simulink library "ET3036TU_model_library_2021b"  (R2021b)
settings: Solver=VariableStepAuto  StartTime=0.0  StopTime=10.0  RelTol=1e-3
values from neighbouring files (symbols this model uses):
  Data =     [Data.mat]
  E_tol = 100    [run_test.m]
  Fnom = 50    [run_test.m]
  OverChargingProtection = 0    [run_test.m]
  simulation_mode = 2    [run_test.m]
  T_err = 60*60    (= 3600)    [run_test.m]
  Tsample = 60    [run_test.m]
  Vnom = sqrt(3)*230    [run_test.m]
undefined symbols (not defined in the file or in its folder): sigbuilder_block, sim_text
libraries: simulink x13, spsThreePhaseDynamicLoadLib x5, spsPower3phPhasorLib x3, eePowerMeasurement x2, spsThreePhaseVIMeasurementLib x2, spsThreePhaseSourceLib x2, spspowerguiLib x2, spsPower3phInstantaneousLib x1, spsThreePhaseSeriesRLCLoadLib x1, $bdroot x1
(part 1 of 2)
Description:
  | The following SIMULINK library is designed for the course "ET3036TU- PROJECT DESIGN FOR SUSTAINABLE ENERGY SYSTEMS". This is offered by EEMCS, TU Delft.
  | The following library was originally developed in R2020a and updated to 2020b. Contributors: N. K. Panda (n.k.panda@tudelft.nl), Simon Tindemans (s.h.tindemans@tudelft.nl)
settings Model: ModifiedComment=nkpanda -- 14 Nov 14:41:00 2023 -- Version2023.1 -- Updated to 2023b  Creator=Hazem  LastModifiedBy=nkpanda
settings Model: ModifiedHistory=|
  | nkpanda -- 14 Nov 14:41:00 2023 -- Version2023.1 -- Updated to 2023b
  | 
  | nkpanda -- Thu Dec 01 18:21:02 2022 -- Version 2.023160e+03 --updated bus meassurement icon
  | 
  | nkpanda -- Thu Dec 01 18:06:26 2022 -- Version 2.023150e+03
  | 
  | nkpanda -- Thu Dec 01 18:02:35 2022 -- Version 2.023140e+03 --renamed V2
  | 
  | nkpanda -- Mon Nov 28 16:04:20 2022 -- Version 2.023100e+03 -- meassurement channel updates
  | 
  | nkpanda -- Mon Nov 28 15:57:43 2022 -- Version 2022.10 (updated bus meassurement)
  | 
  | nkpanda -- Wed Nov 23 09:50:22 2022 -- Version 2.023500e+03
  | 
  | nkpanda -- Wed Nov 23 09:47:48 2022 -- Version 2022_updated_savedparam
  | 
  | nkpanda -- Upload version Tue Nov 15 14:46:24 2022 -- Version 2.022.4
  | 
  | nkpanda -- Tue Nov 15 14:32:50 2022 -- Version 2022.3
  | 
  | nkpanda -- Tue Nov 15 14:15:04 2022 -- Version 2022.2
  | 
  | nkpanda -- Tue Nov 15 13:41:17 2022 -- Version 2022.1
  | 
  | Original version: cc Hazem
  | Lates version : cc nkpanda
settings SolverCC: AlgebraicLoopSolver=TrustRegion
settings DebuggingCC: SFMachineParentedDataDiag=warning  ArithmeticOperatorsInVariantConditions=warning
settings SFSimCC: CustomCodeUndefinedFunction=UseInterfaceOnly

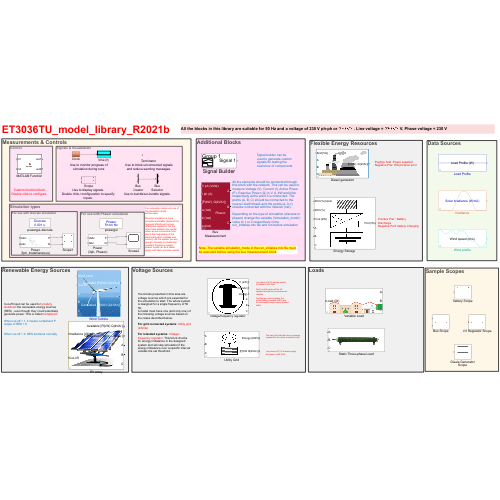
[thumbnail: Simulink's stored preview of the top-level diagram]
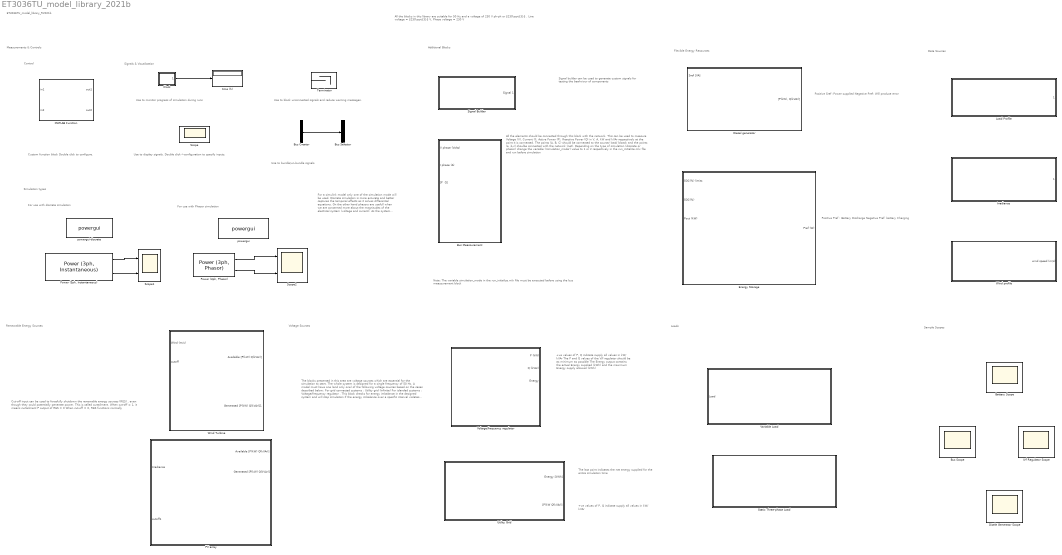
== system ET3036TU_model_library_2021b ==
  note: Note: The variable simulation_mode in the run_initialize.mlx file must be executed before using the bus meassurement block
  note: For a simulink model only one of the simulation mode
      | will be used.
      |
      | Discrete simulation is more accurate and better captures the temporal effects as it solves differential equations. On the other hand phasors are usefull when we are concerned more about the magnitudes of the electrical system (voltage and current). As the system you are going to develop is a balanced constant frequency system, phasor mode can be a faster option with fairly accurate results,
  note: Data Sources
  note: Additional Blocks
  note: Sample Scopes
  note: All the blocks in this library are suitable for 50 Hz and a voltage of 230 V ph-ph or $230\sqrt{3}$ . Line voltage = $230\sqrt{3}$ V, Phase voltage = 230 V
  note: +ve values of P, Q indicate supply
      | all values in kW/ kVAr
      |
      | The P and Q values of the V/f regulator should be as minimum as possible
      |
      | The Energy output contains the actual Energy supplied (kWh) and the maximum Energy supply allowed (kWh)
  note: All the elements should be connected through this block with the network. This can be used to measure Voltage (V), Current (I), Active Power (P), Reactive Power (Q) in V, A, kW and kVAr respectively at the point it is connected. The points (A, B, C) should be connected to the source/ load/ bloack and the points (a ,b,c) shoulbe connected with the network (net).
      |
      | Depending on the type of simulation (discrete or phasor) change the variable ('simulation_mode') value to 1 or 2 respectively in the run_initialize.mlx file and run before simulation
  note: Flexible Energy Resources
  note: Signals & Visualization
  note: Control
  note: Simulation types
  note: ET3036TU_model_library_R2021b
  note: The blocks presented in this area are voltage sources which are essential for the simulation to start. The whole system is designed for a single frequency of 50 Hz.
      | A model must have one (and only one) of the following voltage sources based on the cases described below:
      |
      | For grid connected systems : Utility grid (infinite)
      |
      | For islanded systems : Voltage/frequency regulator . This block checks for energy imbalance in the designed system and will stop simulation if the energy imbalance over a specific interval violates the set threshold.
  note: Loads
  note: Voltage Sources
  note: Custom function block
      | Double click to configure.
  note: Use to display signals.
      | Double click->configuration to specify inputs.
  note: Use to bundle\un-bundle signals.
  note: Use to block unconnected signals
      | and reduce warning messages.
  note: Measurements & Controls
  note: Renewable Energy Sources
  note: For use with Phasor simulation
  note: For use with discrete simulation
  note: Use to monitor progress of
      | simulation during runs
  note: +ve values of P, Q indicate supply
      | all values in kW/ kVAr
  note: The last point indicates the net energy supplied for the entire simulation time
  note: Positive Pref : Battery Discharge
      | Negative Pref: battery Charging
  note: Positive Sref :Power supplied
      | Negative Pref: Will produce error
  note: Signal builder can be used to generate custom signals for testing the beahviour of components
  note: Cut-off input can be used to forcefully shutdown the renewable energy sources (RES) , even though they could potentially generate power. This is called curtailment.
      |
      | When cut-off = 1, it means curtailment P output of RES = 0
      |
      | When cut-off = 0, RES functions normally
  Battery Scope : Scope
  Bus Creator : BusCreator  Inputs=2
  Bus Selector : BusSelector  OutputSignals=Active power P (W),Reactive power Q (var)
  "Bus Meassurement " : Subsystem  mask{SimModeSelect=simulation_mode, dispText=sim_text}
      mask prompts: SimModeSelect "Simulation mode"; dispText "Mode"
      mask init:
      | if SimModeSelect==1
      |     dispText = 'Discrete'
      | elseif SimModeSelect==2
      |     dispText = 'Phasor'
      | end
      mask Display:
      | color('white')
      | port_label('RConn',1,'a (net)')
      | port_label('RConn',2,'b (net)')
      | port_label('RConn',3,'c (net)')
      | port_label('LConn',1,'A')
      | port_label('LConn',2,'B')
      | port_label('LConn',3,'C')
      | 
      | 
      | port_label('output',1,'V ph (Volts)')
      | port_label('output',2,'I ph (A)')
      | port_label('output',3,'[P(kW), Q(kVAr)]')
      | 
      | get_param(gcb,'dispText')
      | 
      | fid = 'ssss'
      | fprintf('            %s \n \n \n \n ',dispText)
  Bus Scope : Scope  NumInputPorts=2
  Clock : Subsystem
  Diesel generator : Subsystem  mask(Controllable Power Plant){Snom=10, Vnom=Vnom, fnom=Fnom, Pfactor=1}
      mask prompts: Snom "Rated Power (kVA)"; Vnom "Rated Line  voltage (Vrms)"; fnom "Frequency (Hz)"; Pfactor "Power Factor (leading)"
      mask help: Implements a controllable (dispatchable) power plant with the required governer and excitation subsystems.
      mask Display: image('$imagefile'); % Use "Edit Image" on toolstrip to change.
  Disele Generator Scope : Scope
  Energy Storage : Subsystem  mask(Grid-connected Energy Storage (PQ Model)){Vn=Vnom, Fn=Fnom, PnomkW=10, kWh_Rated=1, Efficiency=100, LimitVec=[90 10], RechargeSOC=50, Precharge=100, autoRecharge=off, Initial_kWh_pc=35, PQvec=[0 0], ovrchargpro=OverChargingProtection}
      mask prompts: Vn "Nominal Line Voltage [Vrms]"; Fn "Nominal Frequency [Hz]"; PnomkW "Rated Power [kW]"; kWh_Rated "Rated Capacity [kWh]"; Efficiency "Overall System Efficiency [%]"; LimitVec "Upper/Lower Charge Limits [%]"; RechargeSOC "SOC to Recharge [%]"; Precharge "Recharge Rate [% of Rated Power]"; autoRecharge "Enable Auto-Recharge"; Initial_kWh_pc "Initial State-of-Charge [0-100%]"; PQvec "Initial Active/Reactive Cmds"; ovrchargpro "Enable over charging/ discharging protection (0: Disable, 1: Enable)"
      mask help:
      | The energy storage block models a generic grid-connected energy storage system (ESS), most commonly a battery system. This is a system-level model that does not contain any power electronics, but is useful for load flow, phasor, and hybrid phasor-EMT simulations. The inputs to this block are the commanded active and reactive power of the ESS.
      |
      | Note: Positive cmd indicates discharging (supply), negative cmd indicates charging (load).
      | Note: The initial active/reactive power commands must be specified for use for Load Flow analysis.
      mask init:
      | % Calculate Initial Conditions
      | Pnom = PnomkW*1e3;
      | P0 = -PQvec(1);  Q0 = -PQvec(2);
      | if abs(P0) > Pnom
      |     P0 = sign(P0)*Pnom;
      | end
      | 
      | % Calculate Q0 given Reactive Power Capability Curve
      | Qlim = sqrt(Pnom^2 - P0^2);
      | if Qlim > abs(Q0)
      |     Q0 = sign(Q0)*Qlim;
      | end
      | 
      | UpChrgLim = LimitVec(1);
      | LowChrgLim = LimitVec(2);
      | if Initial_kWh_pc > UpChrgLim && P0 < 0
      |     P0 = 0; Q0 = 0;
      | elseif Initial_kWh_pc < LowChrgLim && P0 > 0
      |     P0 = 0; Q0 = 0;
      | end
      mask DialogControl Container7 Prompt: Grid Connection Properties
      mask DialogControl Container11 Prompt: Charge/Discharge Controls
      mask DialogControl Container12 Prompt: Initial Conditions
      mask Display: image('$imagefile'); % Use "Edit Image" on toolstrip to change.
  Irradiance : Subsystem  mask(Irradiance profile){}
      mask help:
      | Automatically loads irradiance values from the local file 'Data.mat' (variable Data.solar).
      |
      | Expects hourly input irradiance values (W/m2).
      mask init:
      | load Data
      mask Display:
      | plot(Data.solar.hour(1:24),Data.solar.direct(1:24)+Data.solar.diffuse(1:24))
      | 
      | color('blue')
      | disp('Solar Irradiance (W/m2)')
  Load Profile : Subsystem
      mask init:
      | load Data
      mask DialogControl DescGroupVar Prompt: Load Profile
      mask DialogControl DescTextVar Prompt: Automatically loads Consumption values from the local file 'Data.mat' (variable Data.varload).
      mask DialogControl Control2 Prompt: Expects per-minute active power consumption values (W).
      mask Display:
      | plot(Data.varload.minute(120:150),Data.varload.load(120:150))
      | color('black')
      | disp('Load Profile (W)')
  MATLAB Function : MATLAB Function  TreatAsAtomicUnit=on
  "PV array " : Subsystem  mask(PV farm){Efficiency=0.2, Area=100, Vnom=Vnom, fnom=Fnom}
      mask prompts: Efficiency "Total efficiency (fraction)"; Area "Area (m2)"; Vnom "Rated Line voltage (Vrms)"; fnom "Rated frequency (Hz):"
      mask help: The product of the efficiency, the area covered by the PV farm and the irradiance in W/m2 will give you the power generated by the PV farm.
      mask Display:
      | color('white')
      | image(imread('pv.jpg'))
      | 
      | color('black')
      | port_label('RConn',1,'A')
      | port_label('RConn',2,'B')
      | port_label('RConn',3,'C')
      | port_label('output',1,'Available [P(kW) Q(kVAr)]')
      | port_label('output',2,'Generated [P(kW) Q(kVAr)]')
      | 
      | port_label('input',1,'Irradiance (W/m2)')
      | port_label('input',2,'Cut-off')
  "Power (3ph, Instantaneous)" : spsPower3phInstantaneousLib/Power (3ph, Instantaneous)
  "Power (3ph, Phasor)" : spsPower3phPhasorLib/Power (3ph, Phasor)
      settings: SourceProductBaseCode=PS
  Scope : Scope  NumInputPorts=2
  Scope1 : Scope  NumInputPorts=2
  Scope2 : Scope  NumInputPorts=2
  Signal Builder : Subsystem  Tag=STV Subsys  LoadFcn=sigbuilder_block('load');  StartFcn=sigbuilder_block('start');  StopFcn=sigbuilder_block('stop');  ClipboardFcn=sigbuilder_block('clipboard');  mask(Sigbuilder block){tuvar=[0:10]}
      mask help: Simulink:masks:SigbuilderBlock_MD
      mask init:
      | if ~strcmp(get_param(bdroot(gcbh),'SimulationStatus'),'stopped') tuvar = sigbuilder_block('maskInit'); end
      settings: CopyFcn=sigbuilder_block('copy');  DeleteFcn=sigbuilder_block('delete');  ModelCloseFcn=sigbuilder_block('modelClose');  PreSaveFcn=sigbuilder_block('preSave');  PauseFcn=sigbuilder_block('pause');  ContinueFcn=sigbuilder_block('continue');  NameChangeFcn=sigbuilder_block('namechange');  OpenFcn=sigbuilder_block('open',[437.6 199.2 550.4 400 ]);  CloseFcn=sigbuilder_block('close');
      mask Display: plot(0, 0, 100, 100,[2, 2, 32, 32, 2], [68, 8, 8, 68, 68],[32, 2], [38, 38], [32, 19, 2],[53, 60, 44], [32, 17, 17, 2],[16, 16, 31, 31]);txt = getActiveGroup(gcbh);text(2, 100, txt,'verticalAlignment', 'top');
  Static Three-phase Load : Subsystem  mask(Static Three-phase Load){Vnom=Vnom, fnom=Fnom, Prated=10}
      mask prompts: Vnom "Nominal Line Voltage Vn (Vrms)"; fnom "Nominal frequency fn (Hz):"; Prated "Active power P (kW):"
      mask help:
      | Implements a three-phase resistive load.
      |
      | Adjust nominal voltage and frequency according to system configuration.
      |
      | Specify rated power consumption.
      mask Display: image(imread('Res.jpg'))
  Terminator : Terminator
  Utility Grid : Subsystem  mask(Utility Distribution Substation){Vnommask=Vnom, Fnommask=Fnom}
      mask prompts: Vnommask "Grid Line voltage (Vrms)"; Fnommask "Nominal frequency (Hz):"
      mask help:
      | Implements a grid connection with finite capacity.
      |
      | Supports two-way power flow, set voltages and frequency according to system configuration.
      |
      | Adjust Nominal Power.
      mask Display: image('$imagefile'); % Use "Edit Image" on toolstrip to change.
  V/f Regulator Scope : Scope
  Variable Load : Subsystem  mask(Variable Load (PQ Model)){Vn=Vnom, Fn=Fnom, PF=1, Load0=0}
      mask prompts: Vn "Nominal Line Voltage [Vrms]"; Fn "Nominal Frequency [Hz]"; PF "Power Factor [0 to 1]"; Load0 "Initial Load [W]"
      mask help:
      | The Variable Load block is a lumped approximation for a distribution feeder. For non-unity power factor loads, the input (active power) is scaled accordingly to generate a desired load.
      |
      | Note: The initial input load must be specified for use for Load Flow analysis.
      mask init:
      | P0 = Load0;
      | Q0 = Load0*sqrt(1/PF-1);
      mask Display:
      | image('house.png')
      | color('black')
      | port_label('input',1,'Load (W)')
      | port_label('Rconn',1,'A')
      | port_label('Rconn',2,'B')
      | port_label('Rconn',3,'C')
  Voltage/frequency regulator : Subsystem  mask{E_max=E_tol, Terr=T_err, Vnommask=Vnom, Fnommask=Fnom}
      mask prompts: E_max "Energy error tolerance  (Wh)"; Terr "Error re-set time-period (seconds)"; Vnommask "Nominal Line Voltage (Vrms)"; Fnommask "Nominal Frequency (Hz)"
      mask Display: image('$imagefile'); % Use "Edit Image" on toolstrip to change.
  "Wind Turbine " : Subsystem  mask{Unom=15, Umax=25, Umin=5, Pselect=1: Simple Cubic Power, fnom=Fnom, Vnom=Vnom, Pnom=20, rp=5, Cp=16/27, rho=1.225, Uvec=1:1:30, Pvec=[0,0,0,0,21359.3750000000,58193.5000000000,104316.125000000,157104.500000000,213935.875000000,272187.500000000,329236.625000000,382460.500000000,429236.375000000,466941.500000000,492953.125000000,500000,500000,500000,500000,500000,500000,500000,500000,500000,500000,0,0,0,0,0], Tp=1, Tq=0.1, ReactP=0}
      mask prompts: Unom "Nominal Wind Speed [m/s]"; Umax "Maximum Operating Wind [m/s]"; Umin "Minimum Operating Wind [m/s]"; Pselect "Wind Turbine Power Model"; fnom "Nominal frequency (Hz):"; Vnom "Nominal phae-to-phase voltage (Vrms)"; Pnom "Nominal Power, [kW]"; rp "Blade Radius, r [m]"; Cp "Performance Coefficient, Cp"; rho "Air Density, rho [kg/m^3]"; Uvec "Wind Vec [m/s]"; Pvec "Power Vec [W]"; Tp "Active Power Dynamics, Tp [s]"; Tq "Reactive Power Dynamics, Tq [s]"; ReactP "Reactive Power Percentage [%]"
      mask help:
      | Simple Wind Turbine that serves as an Active and Reactive Power Source depending on the Wind Power Curve.
      |
      | The Wind Turbine Power Curve can be defined by one of three models:
      | 1: Simple cubic power curve
      | 2: Physical wind turbine parameters
      | 3: Look-up table (from a wind turbine data sheet).
      |
      | Cutoff takes value 1 or 0. 1 denotes manual forced cut-off od wind power generation even though potnetial wind power is available
      | The 'General' and 'Dynamics' tabs apply to all models.
      mask init:
      | A = pi*rp^2;
      | 
      | if Pselect == 1,
      |     Pmax = Pnom*1e3;
      | elseif Pselect == 2,
      |     Pmax = 1/2*rho*Cp*A*Umax^3;
      | else
      |     Pmax = max(Pvec);
      | end
      | Qmax = (ReactP/100)*Pmax;
      mask TypeOptions Pselect: 1: Simple Cubic Power | 2: Physical parameters | 3: Look-up Fit
      mask DialogControl Container4 Prompt: General
      mask DialogControl Container16 Prompt: Turbine
      mask DialogControl Container10 Prompt: Electrical
      mask DialogControl Container12 Prompt: 1: Cubic
      mask DialogControl Container9 Prompt: 2: Physical
      mask DialogControl Container7 Prompt: 3: Lookup
      mask DialogControl Container8 Prompt: Dynamics
      mask Display:
      | image(imread('eolienne.bmp'))
      | 
      | color('white')
      | port_label('LConn',1,'A')
      | port_label('LConn',2,'B')
      | port_label('LConn',3,'C')
      | 
      | port_label('output',1,'Available [P(kW) Q(kVAr)]')
      | port_label('output',2,'Generated [P(kW) Q(kVAr)]')
      | port_label('input',1,'Wind (m/s)')
      | port_label('input',2,'Cut-off')
  Wind profile : Subsystem  mask(Wind profile){}
      mask help:
      | Automatically loads wind speeds from the local file 'Data.mat' (variable Data.wind).
      |
      | Expects hourly input wind speeds (m/s).
      mask init:
      | load Data
      mask Display:
      | plot(Data.wind.hour(1:24),Data.wind.speed(1:24))
      | color('black')
      | disp('Wind speed (m/s)')
  powergui : spspowerguiLib/powergui  Priority=1  SimulationMode=Phasor  SampleTime=50e-6  frequency=Fnom  Iterations=50  frequencyindice=60  Pbase=100e6  ErrMax=1e-4  UnitsV=kV  UnitsW=MW  buscounter=0  FunctionMessages=off  echomessages=off  EnableUseOfTLC=off  CurrentSourceSwitches=off  DisableSnubberDevices=off  DisableRonSwitches=off  DisableVfSwitches=off  DisplayEquations=off  AutomaticDiscreteSolvers=off  SolverType=Tustin/Backward Euler (TBE)  Interpol=off  ExternalGateDelay=off  methode=off  Ts=100  x0status=blocks  SPID=on  SwTol=0  HookPort=off  NonlinearTolerance=1e-4  nMaxIteration=100  ContinueOnMaxIteration=off  RestoreLinks=warning  ResistiveCurrentMeasurement=off  Frange=[0:2:500]  Ylog=off  Xlog=on  ShowGrid=off  save=off  variable=ZData  structure=0  ZoomFFT=off  StartTime=0.0  cycles=1  DisplayStyle=1  fundamental=60  FreqAxis=off  MaxFrequency=1000  frequencyindicesteady=1  RmsSteady=1  display=off
  powergui-discrete : spspowerguiLib/powergui  Priority=1  SimulationMode=Discrete  SampleTime=1e-3  frequency=60  Iterations=50  frequencyindice=60  Pbase=100e6  ErrMax=1e-4  UnitsV=kV  UnitsW=MW  buscounter=0  FunctionMessages=off  echomessages=off  EnableUseOfTLC=off  CurrentSourceSwitches=off  DisableSnubberDevices=off  DisableRonSwitches=off  DisableVfSwitches=off  DisplayEquations=off  AutomaticDiscreteSolvers=off  SolverType=Tustin/Backward Euler (TBE)  Interpol=off  ExternalGateDelay=off  methode=off  Ts=100  x0status=blocks  SPID=on  SwTol=0  HookPort=off  NonlinearTolerance=1e-4  nMaxIteration=100  ContinueOnMaxIteration=off  RestoreLinks=warning  ResistiveCurrentMeasurement=off  Frange=[0:2:500]  Ylog=off  Xlog=on  ShowGrid=off  save=off  variable=ZData  structure=0  ZoomFFT=off  StartTime=0.0  cycles=1  DisplayStyle=1  fundamental=60  FreqAxis=off  MaxFrequency=1000  frequencyindicesteady=1  RmsSteady=1  display=off
  time (h) : Display
      settings: Format=bank
  wires:
  "Power (3ph, Phasor)"/1 -> Scope2/1
  "Power (3ph, Phasor)"/2 -> Scope2/2
  "Power (3ph, Instantaneous)"/1 -> Scope1/1
  "Power (3ph, Instantaneous)"/2 -> Scope1/2
  Clock/1(" ") -> time (h)/1
  Bus Creator/1 -> Bus Selector/1

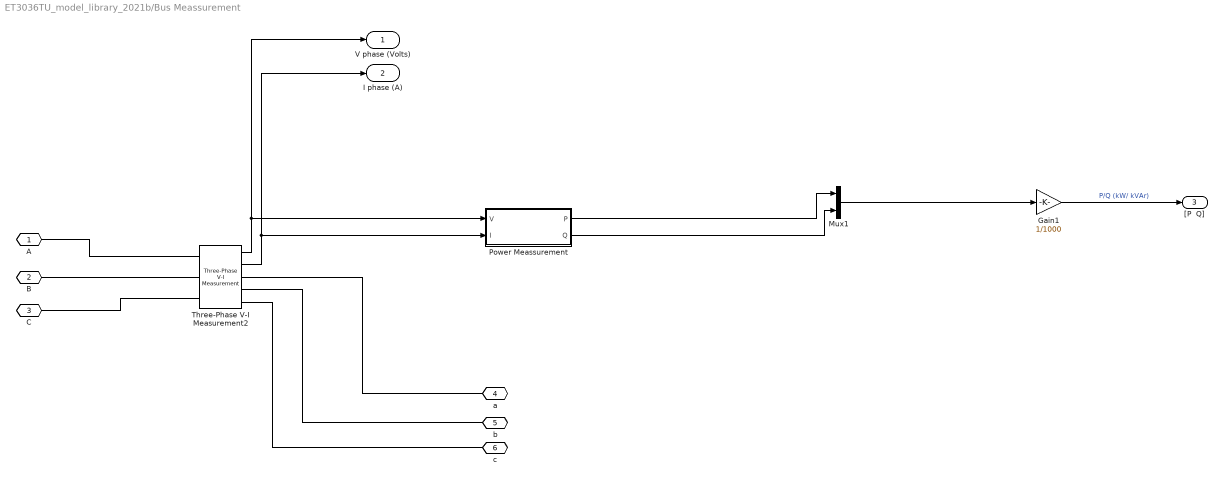
== system ET3036TU_model_library_2021b/Bus Meassurement  ==
  Gain1 : Gain  Gain=1/1000
  Mux1 : Mux  Inputs=2
  Power Meassurement : Subsystem  Variant=on
  Three-Phase V-I Measurement2 : spsThreePhaseVIMeasurementLib/Three-Phase V-I Measurement  VoltageMeasurement=phase-to-ground  SetLabelV=off  LabelV=Vabc  Vpu=off  VpuLL=off  CurrentMeasurement=yes  SetLabelI=off  LabelI=Iabc  Ipu=off  Pbase=100e6  Vbase=500e3  OutputType=Complex  PhasorSimulation=off  PSBequivalent=0
  A : PMIOPort  Side=Left
  B : PMIOPort  Port=2  Side=Left
  C : PMIOPort  Port=3  Side=Left
  a : PMIOPort  Port=4  Side=Right
  b : PMIOPort  Port=5  Side=Right
  c : PMIOPort  Port=6  Side=Right
  V phase (Volts) : Outport
  I phase (A) : Outport  Port=2
  "[P  Q]" : Outport  Port=3
  wires:
  Gain1/1 -> "[P  Q]"/1  "P/Q (kW/ kVAr)"
  Mux1/1 -> Gain1/1
  Three-Phase V-I Measurement2/2 -> I phase (A)/1, Power Meassurement/2(I)
  Three-Phase V-I Measurement2/1 -> V phase (Volts)/1, Power Meassurement/1(V)
  Power Meassurement/2(Q) -> Mux1/2
  Power Meassurement/1(P) -> Mux1/1
  connections:
  Three-Phase V-I Measurement2/LConn3 -- C/RConn1
  B/RConn1 -- Three-Phase V-I Measurement2/LConn2
  A/RConn1 -- Three-Phase V-I Measurement2/LConn1
  Three-Phase V-I Measurement2/RConn1 -- a/RConn1
  Three-Phase V-I Measurement2/RConn2 -- b/RConn1
  Three-Phase V-I Measurement2/RConn3 -- c/RConn1

== system ET3036TU_model_library_2021b/Clock ==
  Clock : Clock
  Gain : Gain  Gain=1/(60*60)
  " " : Outport  VectorParamsAs1DForOutWhenUnconnected=off
  wires:
  Gain/1 -> " "/1
  Clock/1 -> Gain/1

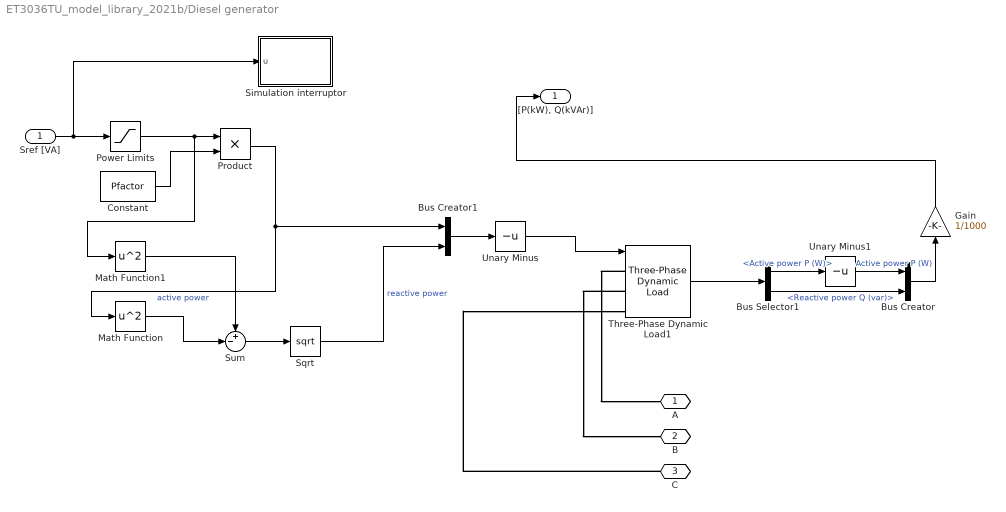
== system ET3036TU_model_library_2021b/Diesel generator ==
  Sref [VA] : Inport
  Bus Creator : BusCreator  Inputs=2
  Bus Creator1 : BusCreator  Inputs=2
  Bus Selector1 : BusSelector  OutputSignals=Active power P (W),Reactive power Q (var)
  Constant : Constant  Value=Pfactor
  Gain : Gain  Gain=1/1000
  Math Function : Math  Operator=square  SignedPower=on  SaturateOnIntegerOverflow=on
  Math Function1 : Math  Operator=square  SignedPower=on  SaturateOnIntegerOverflow=on
  Power Limits : Saturate  UpperLimit=Snom*1e3  LowerLimit=0
  Product : Product
  Simulation interruptor : MATLAB Function  TreatAsAtomicUnit=on
  Sqrt : Sqrt  SaturateOnIntegerOverflow=on
  Sum : Sum  Inputs=+-|
  Three-Phase Dynamic Load1 : spsThreePhaseDynamicLoadLib/Three-Phase Dynamic Load  NominalVoltage=[Vnom fnom]  ActiveReactivePowers="[ 0  0]"  PositiveSequence=[Vnom 0]  ExternalControl=on  NpNq=[1.3 2]  TimeConstants="[0  0  0  0]"  MinimumVoltage=0.7  Tfilter=1e-4  LoadFlowParameters=[4,0,0,0,0]
      settings: SourceProductBaseCode=PS
  Unary Minus : UnaryMinus
  Unary Minus1 : UnaryMinus
  A : PMIOPort  Side=Left
  B : PMIOPort  Port=2  Side=Left
  C : PMIOPort  Port=3  Side=Left
  "[P(kW), Q(kVAr)]" : Outport  VectorParamsAs1DForOutWhenUnconnected=off
  wires:
  Gain/1 -> "[P(kW), Q(kVAr)]"/1
  Constant/1 -> Product/2
  Math Function1/1 -> Sum/1
  Math Function/1 -> Sum/2
  Product/1 -> Math Function/1, Bus Creator1/1  "active power"
  Sref [VA]/1 -> Power Limits/1, Simulation interruptor/1(u)
  Sum/1 -> Sqrt/1
  Power Limits/1 -> Math Function1/1, Product/1
  Sqrt/1 -> Bus Creator1/2  "reactive power"
  Bus Selector1/2 -> Bus Creator/2  "<Reactive power Q (var)>"
  Three-Phase Dynamic Load1/1 -> Bus Selector1/1
  Bus Selector1/1 -> Unary Minus1/1  "<Active power P (W)>"
  Unary Minus1/1 -> Bus Creator/1  "Active power P (W)"
  Bus Creator/1 -> Gain/1
  Bus Creator1/1 -> Unary Minus/1
  Unary Minus/1 -> Three-Phase Dynamic Load1/1
  connections:
  C/RConn1 -- Three-Phase Dynamic Load1/LConn3
  Three-Phase Dynamic Load1/LConn2 -- B/RConn1
  Three-Phase Dynamic Load1/LConn1 -- A/RConn1

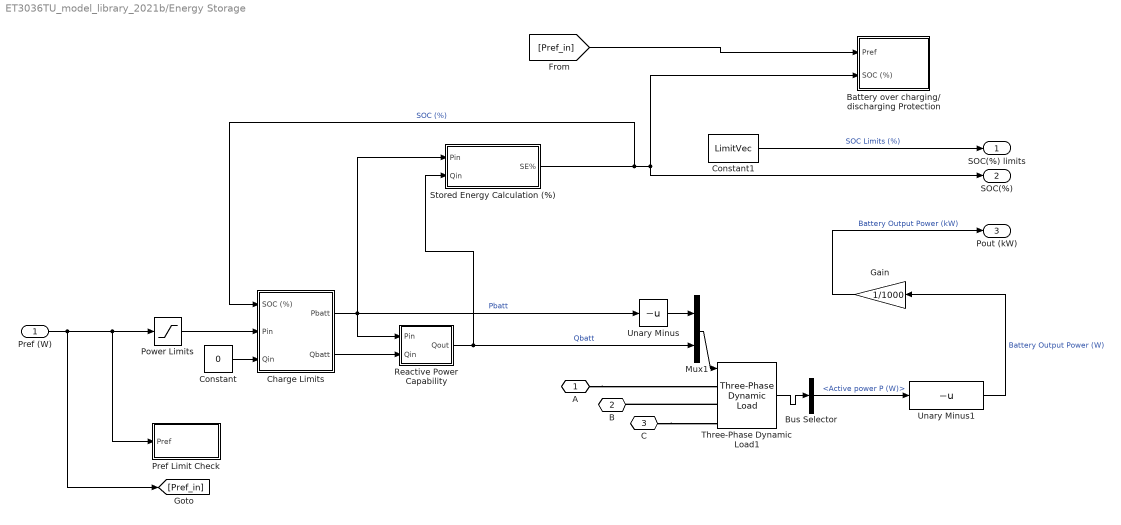
== system ET3036TU_model_library_2021b/Energy Storage ==
  Pref (W) : Inport
  Battery over charging/ discharging Protection : Subsystem
  Bus Selector : BusSelector  OutputSignals=Active power P (W)
  Charge Limits : Subsystem
  Constant : Constant  Value=0
  Constant1 : Constant  Value=LimitVec
  Gain : Gain  Gain=1/1000
  Mux1 : Mux  Inputs=2
  Power Limits : Saturate  UpperLimit=Pnom  LowerLimit=-Pnom
  Pref Limit Check : Subsystem
  Reactive Power Capability : Subsystem
  Stored Energy Calculation (%) : Subsystem
  Three-Phase Dynamic Load1 : spsThreePhaseDynamicLoadLib/Three-Phase Dynamic Load  NominalVoltage=[Vn Fn]  ActiveReactivePowers="[ 0  0]"  PositiveSequence=[Vn 0]  ExternalControl=on  NpNq=[1.3 2]  TimeConstants="[0  0  0  0]"  MinimumVoltage=0.7  Tfilter=1e-4  LoadFlowParameters=[4,0,0,0,0]
      settings: SourceProductBaseCode=PS
  Unary Minus : UnaryMinus
  Unary Minus1 : UnaryMinus
  A : PMIOPort  Side=Right
  B : PMIOPort  Port=2  Side=Right
  C : PMIOPort  Port=3  Side=Right
  SOC(%) limits : Outport  VectorParamsAs1DForOutWhenUnconnected=off
  SOC(%) : Outport  Port=2  VectorParamsAs1DForOutWhenUnconnected=off
  Pout (kW) : Outport  Port=3  VectorParamsAs1DForOutWhenUnconnected=off
  wires:
  Constant1/1 -> SOC(%) limits/1  "SOC Limits (%)"
  [Pref_in] -> Battery over charging/ discharging Protection/1(Pref)
  Gain/1 -> Pout (kW)/1  "Battery Output Power (kW)"
  Unary Minus1/1 -> Gain/1  "Battery Output Power (W)"
  Bus Selector/1 -> Unary Minus1/1  "<Active power P (W)>"
  Charge Limits/2(Qbatt) -> Reactive Power Capability/2(Qin)
  Constant/1 -> Charge Limits/3(Qin)
  Power Limits/1 -> Charge Limits/2(Pin)
  Charge Limits/1(Pbatt) -> Reactive Power Capability/1(Pin), Unary Minus/1, Stored Energy Calculation (%)/1(Pin)  "Pbatt"
  Stored Energy Calculation (%)/1(SE%) -> Charge Limits/1(SOC (%)), SOC(%)/1, Battery over charging/ discharging Protection/2(SOC (%))  "SOC (%)"
  Pref (W)/1 -> Power Limits/1, Pref Limit Check/1(Pref), [Pref_in]
  Reactive Power Capability/1(Qout) -> Mux1/2, Stored Energy Calculation (%)/2(Qin)  "Qbatt"
  Three-Phase Dynamic Load1/1 -> Bus Selector/1
  Mux1/1 -> Three-Phase Dynamic Load1/1
  Unary Minus/1 -> Mux1/1
  connections:
  A/RConn1 -- Three-Phase Dynamic Load1/LConn1
  C/RConn1 -- Three-Phase Dynamic Load1/LConn3
  Three-Phase Dynamic Load1/LConn2 -- B/RConn1

== system ET3036TU_model_library_2021b/Irradiance ==
  Add : Sum
  Add1 : Sum
  Clock1 : Clock
  Constant1 : Constant
  Diffuse irradiance series : Lookup_n-D  NumberOfTableDimensions=1  BreakpointsForDimension1=Data.solar.hour  BeginIndexSearchUsingPreviousIndexResult=on  Table=Data.solar.diffuse  InternalRulePriority=Speed  RndMeth=Simplest  InputSameDT=on
  Direct irradiance series : Lookup_n-D  NumberOfTableDimensions=1  BreakpointsForDimension1=Data.solar.hour  BeginIndexSearchUsingPreviousIndexResult=on  Table=Data.solar.direct  InternalRulePriority=Speed  RndMeth=Simplest  InputSameDT=on
  Second-->Hour : Gain  Gain=1/(60*60)
  " " : Outport  VectorParamsAs1DForOutWhenUnconnected=off
  wires:
  Constant1/1 -> Add/2
  Add/1 -> Direct irradiance series/1, Diffuse irradiance series/1  "Simulation hour"
  Clock1/1 -> Second-->Hour/1
  Second-->Hour/1 -> Add/1
  Diffuse irradiance series/1 -> Add1/1
  Direct irradiance series/1 -> Add1/2
  Add1/1 -> " "/1  "Simulation hour"

== system ET3036TU_model_library_2021b/Load Profile ==
  Add : Sum
  Clock1 : Clock
  Constant1 : Constant
  Second-->Minute : Gain  Gain=1/(60)
  load profile series : Lookup_n-D  NumberOfTableDimensions=1  BreakpointsForDimension1=Data.varload.minute  BeginIndexSearchUsingPreviousIndexResult=on  Table=Data.varload.load  InternalRulePriority=Speed  RndMeth=Simplest  InputSameDT=on
  " " : Outport  VectorParamsAs1DForOutWhenUnconnected=off
  wires:
  Constant1/1 -> Add/2
  Add/1 -> load profile series/1  "Minute"
  load profile series/1 -> " "/1
  Clock1/1 -> Second-->Minute/1
  Second-->Minute/1 -> Add/1

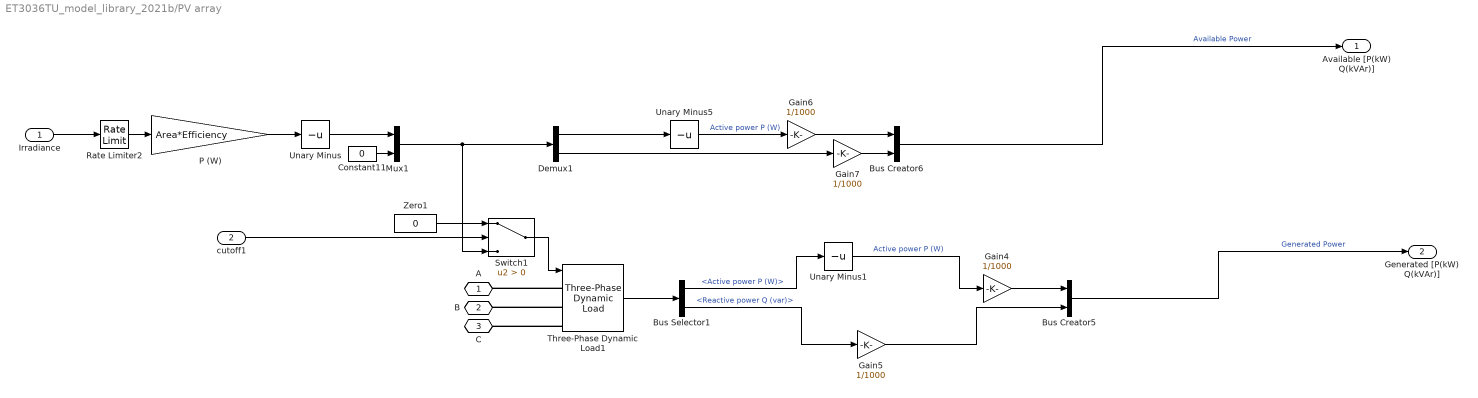
== system ET3036TU_model_library_2021b/PV array  ==
  Irradiance : Inport
  cutoff1 : Inport  Port=2
  Bus Creator5 : BusCreator  Inputs=2
  Bus Creator6 : BusCreator  Inputs=2
  Bus Selector1 : BusSelector  OutputSignals=Active power P (W),Reactive power Q (var)
  Constant11 : Constant  Value=0
  Demux1 : Demux  Outputs=2
  Gain{4..7} (4 alike) : Gain  Gain=1/1000
  Mux1 : Mux  Inputs=2
  P (W) : Gain  Gain=Area*Efficiency
  Rate Limiter2 : RateLimiter  RisingSlewLimit=1e4  FallingSlewLimit=-1e4  SampleTimeMode=inherited
  Switch1 : Switch  Criteria=u2 > Threshold
  Three-Phase Dynamic Load1 : spsThreePhaseDynamicLoadLib/Three-Phase Dynamic Load  NominalVoltage=[Vnom fnom]  ActiveReactivePowers="[ 0  0]"  PositiveSequence=[Vnom 0]  ExternalControl=on  NpNq=[1.3 2]  TimeConstants="[0  0  0  0]"  MinimumVoltage=0.7  Tfilter=1e-4  LoadFlowParameters=[4,0,0,0,0]
      settings: SourceProductBaseCode=PS
  Unary Minus : UnaryMinus
  Unary Minus1 : UnaryMinus
  Unary Minus5 : UnaryMinus
  Zero1 : Constant  Value=0  OutDataTypeStr=Inherit: Inherit via back propagation
  A : PMIOPort  Side=Right
  B : PMIOPort  Port=2  Side=Right
  C : PMIOPort  Port=3  Side=Right
  Available [P(kW) Q(kVAr)] : Outport  VectorParamsAs1DForOutWhenUnconnected=off
  Generated [P(kW) Q(kVAr)] : Outport  Port=2  VectorParamsAs1DForOutWhenUnconnected=off
  wires:
  Zero1/1 -> Switch1/1
  cutoff1/1 -> Switch1/2
  Mux1/1 -> Switch1/3, Demux1/1
  Switch1/1 -> Three-Phase Dynamic Load1/1
  Bus Creator6/1 -> Available [P(kW) Q(kVAr)]/1  "Available Power"
  Gain7/1 -> Bus Creator6/2
  Unary Minus5/1 -> Gain6/1  "Active power P (W)"
  Demux1/2 -> Gain7/1
  Gain6/1 -> Bus Creator6/1
  Demux1/1 -> Unary Minus5/1
  Gain5/1 -> Bus Creator5/2
  Gain4/1 -> Bus Creator5/1
  Bus Selector1/2 -> Gain5/1  "<Reactive power Q (var)>"
  Three-Phase Dynamic Load1/1 -> Bus Selector1/1
  Unary Minus1/1 -> Gain4/1  "Active power P (W)"
  Bus Selector1/1 -> Unary Minus1/1  "<Active power P (W)>"
  Irradiance/1 -> Rate Limiter2/1
  P (W)/1 -> Unary Minus/1
  Unary Minus/1 -> Mux1/1
  Constant11/1 -> Mux1/2
  Rate Limiter2/1 -> P (W)/1
  Bus Creator5/1 -> Generated [P(kW) Q(kVAr)]/1  "Generated Power"
  connections:
  Three-Phase Dynamic Load1/LConn3 -- C/RConn1
  Three-Phase Dynamic Load1/LConn1 -- A/RConn1
  Three-Phase Dynamic Load1/LConn2 -- B/RConn1

== system ET3036TU_model_library_2021b/Signal Builder ==
  Demux : Demux  Tag=STV Demux  Outputs=1
      settings: DisplayOption=none
  FromWs : FromWorkspace  Tag=STV FromWs  VariableName=tuvar
      SigBuilderData=|
      | common.afterFinalStr = 'Extrapolate'
      | common.sampleTime = 0
      | dataSet.timeRange = [0 10]
      | dataSet.name = 'Group 1'
      | sbobj.Groups.Name = 'Group 1'
      | sbobj.Groups.Signals.Name = 'Signal 1'
      | sbobj.Groups.Signals.XData = [0 4 4 6 6 10]
      | sbobj.Groups.Signals.YData = [0 0 1 1 0 0]
  Signal 1 : Outport  Tag=STV Outport
  wires:
  Demux/1 -> Signal 1/1
  FromWs/1 -> Demux/1

== system ET3036TU_model_library_2021b/Static Three-phase Load ==
  Three-Phase Series RLC Load : spsThreePhaseSeriesRLCLoadLib/Three-Phase Series RLC Load  LConnTagsString=A|B|C  Configuration=Y (grounded)  NominalVoltage=Vnom  Vabc=[1e3 1e3 1e3]  Vabcp=[1e3 1e3 1e3]  NominalFrequency=fnom  UnbalancedPower=off  ActivePower=Prated*1e3  InductivePower=100  CapacitivePower=100  Pabc=[10e3 9e3 11e3]  QLabc=[100 90 110]  QCabc=[100 90 110]  Pabcp=[10e3 9e3 11e3]  QLabcp=[100 90 110]  QCabcp=[100 90 110]  Measurements=None  LoadType=constant Z
  A : PMIOPort  Side=Left
  B : PMIOPort  Port=2  Side=Left
  C : PMIOPort  Port=3  Side=Left
  connections:
  Three-Phase Series RLC Load/LConn2 -- B/RConn1
  C/RConn1 -- Three-Phase Series RLC Load/LConn3
  A/RConn1 -- Three-Phase Series RLC Load/LConn1

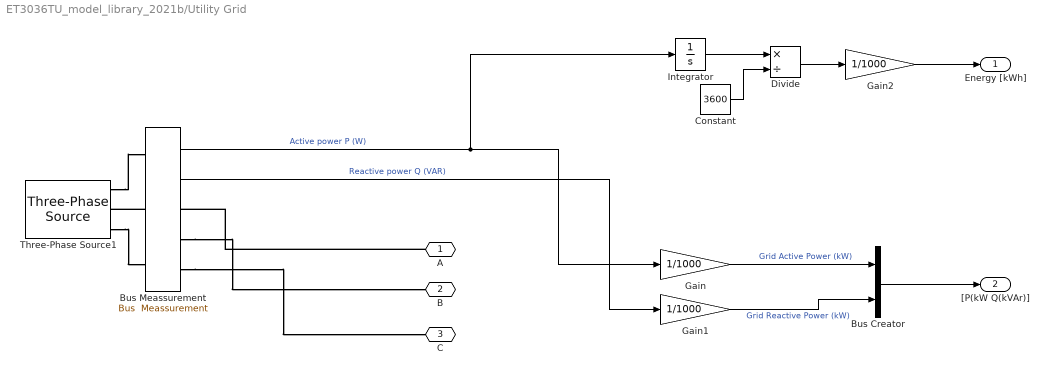
== system ET3036TU_model_library_2021b/Utility Grid ==
  Bus Creator : BusCreator  Inputs=2
  "Bus Meassurement " : $bdroot/Voltage//frequency regulator/Bus  Meassurement 
  Constant : Constant  Value=3600
  Divide : Product  Inputs=*/
  Gain : Gain  Gain=1/1000
  Gain1 : Gain  Gain=1/1000
  Gain2 : Gain  Gain=1/1000
  Integrator : Integrator
  Three-Phase Source1 : spsThreePhaseSourceLib/Three-Phase Source  InternalConnection=Yg  VoltagePhases=off  Voltage=Vnommask  PhaseAngle=0  Voltage_phases=[25e3 25e3 25e3]/sqrt(3)  PhaseAngles_phases=[0 -120 +120]  Frequency=Fnommask  NonIdealSource=off  SpecifyImpedance=off  Resistance=0.8929  Inductance=16.58e-3  ShortCircuitLevel=100e6  BaseVoltage=25e3  XRratio=7  BusType=swing  Pref=10e3  Qref=0  Prefabc=[10e3, 10e3, 10e3]  Qrefabc=[0, 0, 0]  Qmin=-inf  Qmax=inf
  A : PMIOPort  Side=Left
  B : PMIOPort  Port=2  Side=Left
  C : PMIOPort  Port=3  Side=Left
  Energy [kWh] : Outport  VectorParamsAs1DForOutWhenUnconnected=off
  "[P(kW Q(kVAr)]" : Outport  Port=2
  wires:
  Gain/1 -> Bus Creator/1  "Grid Active Power (kW)"
  Bus Creator/1 -> "[P(kW Q(kVAr)]"/1
  Constant/1 -> Divide/2
  Divide/1 -> Gain2/1
  Integrator/1 -> Divide/1
  Gain2/1 -> Energy [kWh]/1
  Gain1/1 -> Bus Creator/2  "Grid Reactive Power (kW)"
  "Bus Meassurement "/1 -> Integrator/1, Gain/1  "Active power P (W)"
  "Bus Meassurement "/2 -> Gain1/1  "Reactive power Q (VAR)"
  connections:
  "Bus Meassurement "/RConn2 -- B/RConn1
  "Bus Meassurement "/RConn3 -- C/RConn1
  "Bus Meassurement "/LConn2 -- Three-Phase Source1/RConn2
  Three-Phase Source1/RConn1 -- "Bus Meassurement "/LConn1
  Three-Phase Source1/RConn3 -- "Bus Meassurement "/LConn3
  A/RConn1 -- "Bus Meassurement "/RConn1

== system ET3036TU_model_library_2021b/Variable Load ==
  Load : Inport
  Dynamic Load Control : Subsystem
  Terminator : Terminator
  Three-Phase Dynamic Load : spsThreePhaseDynamicLoadLib/Three-Phase Dynamic Load  NominalVoltage=[Vn Fn]  ActiveReactivePowers=[0 0]  PositiveSequence=[Vn 0]  ExternalControl=on  NpNq=[1.3 2]  TimeConstants="[0  0  0  0]"  MinimumVoltage=0.7  Tfilter=1e-4  LoadFlowParameters=[4,0,0,0,0]
      settings: SourceProductBaseCode=PS
  A : PMIOPort  Side=Right
  B : PMIOPort  Port=2  Side=Right
  C : PMIOPort  Port=3  Side=Right
  wires:
  Three-Phase Dynamic Load/1 -> Terminator/1
  Dynamic Load Control/1(PQ) -> Three-Phase Dynamic Load/1
  Load/1 -> Dynamic Load Control/1(P0)
  connections:
  A/RConn1 -- Three-Phase Dynamic Load/LConn1
  Three-Phase Dynamic Load/LConn2 -- B/RConn1
  Three-Phase Dynamic Load/LConn3 -- C/RConn1

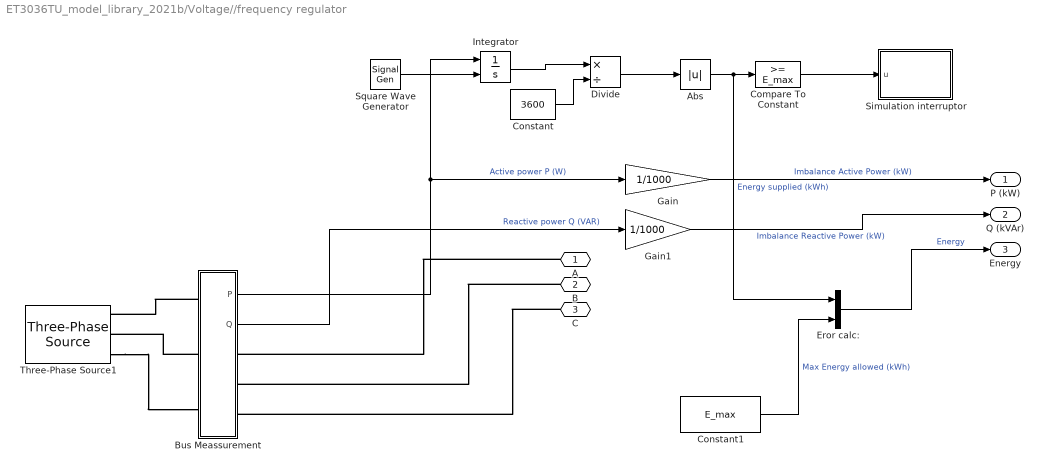
== system ET3036TU_model_library_2021b/Voltage//frequency regulator ==
  Abs : Abs
  "Bus Meassurement " : Subsystem  mask{SimModeSelect=simulation_mode, dispText=sim_text}
      mask prompts: SimModeSelect "Simulation mode"; dispText "Mode"
  Compare To Constant : simulink/Logic and Bit Operations/Compare To Constant  relop=>=  const=E_max  OutDataTypeStr=boolean
  Constant : Constant  Value=3600
  Constant1 : Constant  Value=E_max
  Divide : Product  Inputs=*/
  Eror calc: : Mux  Inputs=2
  Gain : Gain  Gain=1/1000
  Gain1 : Gain  Gain=1/1000
  Integrator : Integrator  ExternalReset=either
  Simulation interruptor : MATLAB Function  TreatAsAtomicUnit=on
  Square Wave Generator : SignalGenerator  WaveForm=square  Frequency=1/(2*Terr)
  Three-Phase Source1 : spsThreePhaseSourceLib/Three-Phase Source  InternalConnection=Yg  VoltagePhases=off  Voltage=Vnommask  PhaseAngle=0  Voltage_phases=[25e3 25e3 25e3]/sqrt(3)  PhaseAngles_phases=[0 -120 +120]  Frequency=Fnommask  NonIdealSource=off  SpecifyImpedance=off  Resistance=0.8929  Inductance=16.58e-3  ShortCircuitLevel=100e6  BaseVoltage=25e3  XRratio=7  BusType=swing  Pref=10e3  Qref=0  Prefabc=[10e3, 10e3, 10e3]  Qrefabc=[0, 0, 0]  Qmin=-inf  Qmax=inf
  A : PMIOPort  Side=Right
  B : PMIOPort  Port=2  Side=Right
  C : PMIOPort  Port=3  Side=Right
  P (kW) : Outport
  Q (kVAr) : Outport  Port=2
  Energy : Outport  Port=3
  wires:
  Constant1/1 -> Eror calc:/2  "Max Energy allowed (kWh)"
  Gain1/1 -> Q (kVAr)/1  "Imbalance Reactive Power (kW)"
  Gain/1 -> P (kW)/1  "Imbalance Active Power (kW)"
  Square Wave Generator/1 -> Integrator/2
  Abs/1 -> Compare To Constant/1, Eror calc:/1  "Energy supplied (kWh)"
  Divide/1 -> Abs/1
  Constant/1 -> Divide/2
  Compare To Constant/1 -> Simulation interruptor/1(u)
  "Bus Meassurement "/2(Q) -> Gain1/1  "Reactive power Q (VAR)"
  Integrator/1 -> Divide/1
  "Bus Meassurement "/1(P) -> Gain/1, Integrator/1  "Active power P (W)"
  Eror calc:/1 -> Energy/1  "Energy"
  connections:
  B/RConn1 -- "Bus Meassurement "/RConn2
  Three-Phase Source1/RConn3 -- "Bus Meassurement "/LConn3
  A/RConn1 -- "Bus Meassurement "/RConn1
  "Bus Meassurement "/LConn2 -- Three-Phase Source1/RConn2
  "Bus Meassurement "/LConn1 -- Three-Phase Source1/RConn1
  C/RConn1 -- "Bus Meassurement "/RConn3

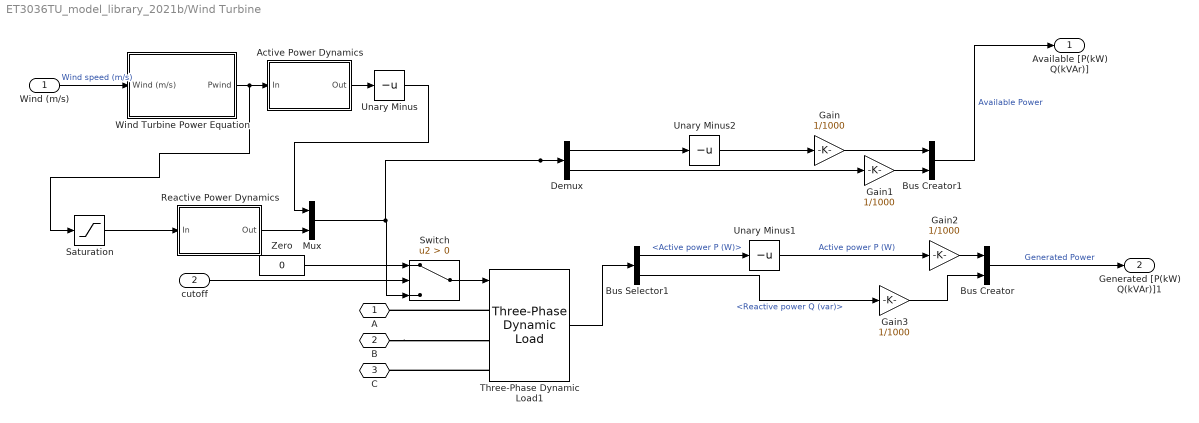
== system ET3036TU_model_library_2021b/Wind Turbine  ==
  Wind (m/s) : Inport
  cutoff : Inport  Port=2
  Active Power Dynamics : Subsystem  VariantControl=T6NotZero
      mask Display: disp('1 / (1 + s T_P)','texmode','on');
  Bus Creator : BusCreator  Inputs=2
  Bus Creator1 : BusCreator  Inputs=2
  Bus Selector1 : BusSelector  OutputSignals=Active power P (W),Reactive power Q (var)
  Demux : Demux  Outputs=2
  Gain{,1..3} (4 alike) : Gain  Gain=1/1000
  Mux : Mux  Inputs=2
  Reactive Power Dynamics : Subsystem  VariantControl=T6NotZero
      mask Display: disp('1 / (1 + s T_Q)','texmode','on');
  Saturation : Saturate  UpperLimit=Qmax  LowerLimit=-Qmax
  Switch : Switch  Criteria=u2 > Threshold
  Three-Phase Dynamic Load1 : spsThreePhaseDynamicLoadLib/Three-Phase Dynamic Load  NominalVoltage=[Vnom fnom]  ActiveReactivePowers="[ 0  0]"  PositiveSequence=[Vnom 0]  ExternalControl=on  NpNq=[1.3 2]  TimeConstants="[0  0  0  0]"  MinimumVoltage=0.7  Tfilter=1e-4  LoadFlowParameters=[4,0,0,0,0]
      settings: SourceProductBaseCode=PS
  Unary Minus : UnaryMinus
  Unary Minus1 : UnaryMinus
  Unary Minus2 : UnaryMinus
  Wind Turbine Power Equation : Subsystem
  Zero : Constant  Value=0  OutDataTypeStr=Inherit: Inherit via back propagation
  A : PMIOPort  Side=Left
  B : PMIOPort  Port=2  Side=Left
  C : PMIOPort  Port=3  Side=Left
  Available [P(kW) Q(kVAr)] : Outport  VectorParamsAs1DForOutWhenUnconnected=off
  Generated [P(kW) Q(kVAr)]1 : Outport  Port=2  VectorParamsAs1DForOutWhenUnconnected=off
  wires:
  Bus Creator/1 -> Generated [P(kW) Q(kVAr)]1/1  "Generated Power"
  Bus Creator1/1 -> Available [P(kW) Q(kVAr)]/1  "Available Power"
  Gain3/1 -> Bus Creator/2
  Gain2/1 -> Bus Creator/1
  Gain1/1 -> Bus Creator1/2
  Gain/1 -> Bus Creator1/1
  Unary Minus2/1 -> Gain/1
  Demux/2 -> Gain1/1
  Demux/1 -> Unary Minus2/1
  Zero/1 -> Switch/1
  cutoff/1 -> Switch/2
  Switch/1 -> Three-Phase Dynamic Load1/1
  Mux/1 -> Switch/3, Demux/1
  Wind (m/s)/1 -> Wind Turbine Power Equation/1(Wind (m/s))  "Wind speed (m/s)"
  Saturation/1 -> Reactive Power Dynamics/1(In)
  Reactive Power Dynamics/1(Out) -> Mux/2
  Wind Turbine Power Equation/1(Pwind) -> Active Power Dynamics/1(In), Saturation/1
  Active Power Dynamics/1(Out) -> Unary Minus/1
  Unary Minus/1 -> Mux/1
  Three-Phase Dynamic Load1/1 -> Bus Selector1/1
  Bus Selector1/1 -> Unary Minus1/1  "<Active power P (W)>"
  Unary Minus1/1 -> Gain2/1  "Active power P (W)"
  Bus Selector1/2 -> Gain3/1  "<Reactive power Q (var)>"
  connections:
  Three-Phase Dynamic Load1/LConn1 -- A/RConn1
  Three-Phase Dynamic Load1/LConn3 -- C/RConn1
  B/RConn1 -- Three-Phase Dynamic Load1/LConn2

== system ET3036TU_model_library_2021b/Wind profile ==
  Add : Sum
  Clock1 : Clock
  Constant1 : Constant
  Second-->Hour : Gain  Gain=1/(60*60)
  Wind speed series : Lookup_n-D  NumberOfTableDimensions=1  BreakpointsForDimension1=Data.wind.hour  BeginIndexSearchUsingPreviousIndexResult=on  Table=Data.wind.speed  ExtrapMethod=Clip  UseLastTableValue=on  InternalRulePriority=Speed  RndMeth=Simplest  InputSameDT=on
  wind speed (m/s) : Outport  VectorParamsAs1DForOutWhenUnconnected=off
  wires:
  Second-->Hour/1 -> Add/1
  Add/1 -> Wind speed series/1
  Constant1/1 -> Add/2
  Clock1/1 -> Second-->Hour/1
  Wind speed series/1 -> wind speed (m/s)/1

== system ET3036TU_model_library_2021b/Bus Meassurement /Power Meassurement ==
  note: 1) Add Subsystem or Model blocks as valid variant choices.
      | 2) You cannot connect blocks at this level. At simulation, connectivity is automatically
      | determined, based on the active variant and port name matching.
  V : Inport
  I : Inport  Port=2
  discrete : Subsystem  VariantControl=simulation_mode==1
  phasor : Subsystem  VariantControl=simulation_mode==2
  P : Outport
  Q : Outport  Port=2

== system ET3036TU_model_library_2021b/Energy Storage/Battery over charging// discharging Protection ==
  Pref : Inport
  SOC (%) : Inport  Port=2
  Over Charging Protection : Subsystem
  Under Charging Protection : Subsystem
  wires:
  Pref/1 -> Over Charging Protection/2(Pref), Under Charging Protection/2(Pref)
  SOC (%)/1 -> Over Charging Protection/1(SOC (%)), Under Charging Protection/1(SOC (%))

== system ET3036TU_model_library_2021b/Energy Storage/Charge Limits ==
  SOC (%) : Inport
  Pin : Inport  Port=2
  Qin : Inport  Port=3
  Overcharge Check : Subsystem
  Undercharge Check : Subsystem
  Pbatt : Outport  VectorParamsAs1DForOutWhenUnconnected=off
  Qbatt : Outport  Port=2  VectorParamsAs1DForOutWhenUnconnected=off
  wires:
  SOC (%)/1 -> Overcharge Check/1(SOC (%)), Undercharge Check/1(SOC (%))
  Undercharge Check/2(Qout) -> Qbatt/1
  Pin/1 -> Overcharge Check/2(Pin)
  Overcharge Check/1(Pout) -> Undercharge Check/2(Pin)
  Qin/1 -> Overcharge Check/3(Qin)
  Undercharge Check/1(Pout) -> Pbatt/1  "Pbatt"
  Overcharge Check/2(Qout) -> Undercharge Check/3(Qin)

== system ET3036TU_model_library_2021b/Energy Storage/Pref Limit Check ==
  Pref : Inport
  Abs1 : Abs
  Constant1 : Constant  Value=PnomkW
  Gain : Gain  Gain=1000
  Simulation Stop : MATLAB Function  TreatAsAtomicUnit=on
  Subtract : Sum  Inputs=+-
  wires:
  Gain/1 -> Subtract/1
  Pref/1 -> Abs1/1
  Constant1/1 -> Gain/1
  Abs1/1 -> Subtract/2
  Subtract/1 -> Simulation Stop/1(u)

== system ET3036TU_model_library_2021b/Energy Storage/Reactive Power Capability ==
  Pin : Inport
  Qin : Inport  Port=2
  Constant : Constant  Value=Pnom
  Math Function : Math  Operator=square  SignedPower=on  SaturateOnIntegerOverflow=on
  Math Function1 : Math  Operator=square  SignedPower=on  SaturateOnIntegerOverflow=on
  Saturation Dynamic : simulink/Discontinuities/Saturation Dynamic  OutMin=[]  OutMax=[]  OutDataTypeStr=Inherit: Same as second input  OutDataType=fixdt(1, 16)  OutScaling=2^-10  DoSatur=off
  Sqrt : Sqrt  SaturateOnIntegerOverflow=on
  Sum : Sum  Inputs=-+|
  Unary Minus : UnaryMinus
  Qout : Outport  VectorParamsAs1DForOutWhenUnconnected=off
  wires:
  Sqrt/1 -> Saturation Dynamic/1, Unary Minus/1
  Math Function1/1 -> Sum/1
  Math Function/1 -> Sum/2
  Constant/1 -> Math Function/1
  Sum/1 -> Sqrt/1
  Unary Minus/1 -> Saturation Dynamic/3
  Saturation Dynamic/1 -> Qout/1
  Pin/1 -> Math Function1/1
  Qin/1 -> Saturation Dynamic/2

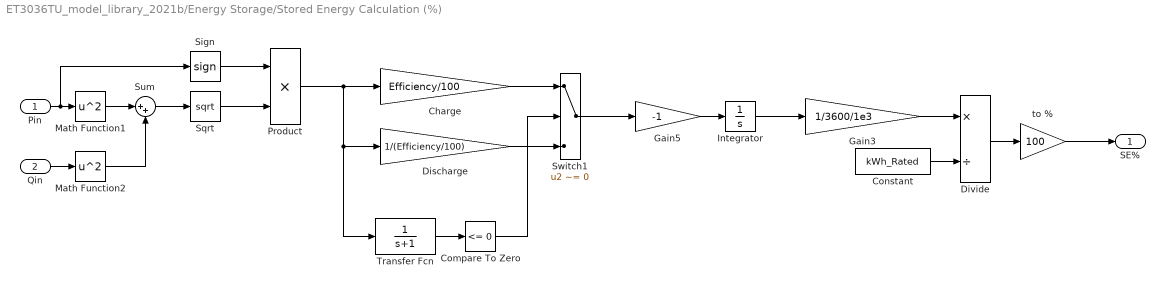
== system ET3036TU_model_library_2021b/Energy Storage/Stored Energy Calculation (%) ==
  Pin : Inport
  Qin : Inport  Port=2
  Charge : Gain  Gain=Efficiency/100
  Compare To Zero : simulink/Logic and Bit Operations/Compare To Zero  relop=<=  OutDataTypeStr=boolean
  Constant : Constant  Value=kWh_Rated
  Discharge : Gain  Gain=1/(Efficiency/100)
  Divide : Product  Inputs=*/
  Gain3 : Gain  Gain=1/3600/1e3
  Gain5 : Gain  Gain=-1
  Integrator : Integrator  InitialCondition=(Initial_kWh_pc/100)*kWh_Rated*3600*1e3
  Math Function1 : Math  Operator=square  SignedPower=on  SaturateOnIntegerOverflow=on
  Math Function2 : Math  Operator=square  SignedPower=on  SaturateOnIntegerOverflow=on
  Product : Product
  Sign : Signum
  Sqrt : Sqrt  SaturateOnIntegerOverflow=on
  Sum : Sum  Inputs=|++
  Switch1 : Switch  Criteria=u2 ~= 0
  Transfer Fcn : TransferFcn  Denominator=[1 1]
  to % : Gain  Gain=100
  SE% : Outport  VectorParamsAs1DForOutWhenUnconnected=off
  wires:
  Sign/1 -> Product/1
  Sqrt/1 -> Product/2
  Sum/1 -> Sqrt/1
  Math Function2/1 -> Sum/2
  Math Function1/1 -> Sum/1
  Qin/1 -> Math Function2/1
  Pin/1 -> Math Function1/1, Sign/1
  Product/1 -> Transfer Fcn/1, Discharge/1, Charge/1
  Discharge/1 -> Switch1/3
  Gain5/1 -> Integrator/1
  to %/1 -> SE%/1
  Transfer Fcn/1 -> Compare To Zero/1
  Switch1/1 -> Gain5/1
  Gain3/1 -> Divide/1
  Constant/1 -> Divide/2
  Charge/1 -> Switch1/1
  Divide/1 -> to %/1
  Compare To Zero/1 -> Switch1/2
  Integrator/1 -> Gain3/1

== system ET3036TU_model_library_2021b/Variable Load/Dynamic Load Control ==
  P0 : Inport
  Fcn : Fcn  Expr=sqrt(1/u(1)-1)
  Mux : Mux  Inputs=2
  Product : Product
  Summer1 : Constant  Value=PF
  PQ : Outport  VectorParamsAs1DForOutWhenUnconnected=off
  wires:
  Product/1 -> Mux/2  "Qo"
  Mux/1 -> PQ/1
  P0/1 -> Mux/1, Product/1
  Fcn/1 -> Product/2
  Summer1/1 -> Fcn/1

== system ET3036TU_model_library_2021b/Voltage//frequency regulator/Bus Meassurement  ==
  Power Meassurement : Subsystem  Variant=on
  Three-Phase V-I Measurement2 : spsThreePhaseVIMeasurementLib/Three-Phase V-I Measurement  VoltageMeasurement=phase-to-ground  SetLabelV=off  LabelV=Vabc  Vpu=off  VpuLL=off  CurrentMeasurement=yes  SetLabelI=off  LabelI=Iabc  Ipu=off  Pbase=100e6  Vbase=500e3  OutputType=Complex  PhasorSimulation=off  PSBequivalent=0
  A : PMIOPort  Side=Left
  B : PMIOPort  Port=2  Side=Left
  C : PMIOPort  Port=3  Side=Left
  a : PMIOPort  Port=4  Side=Right
  b : PMIOPort  Port=5  Side=Right
  c : PMIOPort  Port=6  Side=Right
  P : Outport
  Q : Outport  Port=2
  wires:
  Three-Phase V-I Measurement2/2 -> Power Meassurement/2(I)
  Three-Phase V-I Measurement2/1 -> Power Meassurement/1(V)
  Power Meassurement/1(P) -> P/1
  Power Meassurement/2(Q) -> Q/1
  connections:
  Three-Phase V-I Measurement2/LConn3 -- C/RConn1
  B/RConn1 -- Three-Phase V-I Measurement2/LConn2
  A/RConn1 -- Three-Phase V-I Measurement2/LConn1
  Three-Phase V-I Measurement2/RConn1 -- a/RConn1
  Three-Phase V-I Measurement2/RConn2 -- b/RConn1
  Three-Phase V-I Measurement2/RConn3 -- c/RConn1

== system ET3036TU_model_library_2021b/Wind Turbine /Active Power Dynamics ==
  In : Inport
  1/Tp : Gain  Gain=1/Tp
  Integrator : Integrator
  Sum : Sum  Inputs=|+-
  Out : Outport  VectorParamsAs1DForOutWhenUnconnected=off
  wires:
  Sum/1 -> 1/Tp/1
  1/Tp/1 -> Integrator/1
  In/1 -> Sum/1
  Integrator/1 -> Sum/2, Out/1

== system ET3036TU_model_library_2021b/Wind Turbine /Reactive Power Dynamics ==
  In : Inport
  1/Tq : Gain  Gain=1/Tq
  Integrator : Integrator
  Sum : Sum  Inputs=|+-
  Out : Outport  VectorParamsAs1DForOutWhenUnconnected=off
  wires:
  Integrator/1 -> Out/1, Sum/2
  In/1 -> Sum/1
  1/Tq/1 -> Integrator/1
  Sum/1 -> 1/Tq/1

== system ET3036TU_model_library_2021b/Wind Turbine /Wind Turbine Power Equation ==
  Wind (m/s) : Inport
  Constant : Constant  Value=Pselect
  Cubic Power with Cutoff : Subsystem
  Manufacturer Fit : Lookup_n-D  NumberOfTableDimensions=1  BreakpointsForDimension1=Uvec  Table=Pvec  ExtrapMethod=Clip  InternalRulePriority=Speed  RndMeth=Simplest  InputSameDT=on
  Multiport Switch : MultiPortSwitch
  Saturation : Saturate  UpperLimit=inf  LowerLimit=0  ZeroCross=off
      settings: AttributesFormatString=|
      | %<UpperLimit>
      | %<LowerLimit>
  Wind Turbine Properties : Subsystem
  Pwind : Outport  VectorParamsAs1DForOutWhenUnconnected=off
  wires:
  Cubic Power with Cutoff/1(Pwind) -> Multiport Switch/2
  Wind Turbine Properties/1(Pwind) -> Multiport Switch/3
  Wind (m/s)/1 -> Saturation/1
  Multiport Switch/1 -> Pwind/1
  Constant/1 -> Multiport Switch/1
  Saturation/1 -> Cubic Power with Cutoff/1(Wind (m/s)), Wind Turbine Properties/1(Wind (m/s)), Manufacturer Fit/1
  Manufacturer Fit/1 -> Multiport Switch/4

== system ET3036TU_model_library_2021b/Bus Meassurement /Power Meassurement/discrete ==
  V : Inport
  I : Inport  Port=2
  Power Measurement (Three-Phase) : eePowerMeasurement/Power Measurement (Three-Phase)  LabelModeActiveChoice=Discrete  F=Fnom  K=1  Seq=Positive  Ts=Tsample
      settings: SourceProductBaseCode=PS
  P : Outport
  Q : Outport  Port=2
  wires:
  V/1 -> Power Measurement (Three-Phase)/1
  I/1 -> Power Measurement (Three-Phase)/2
  Power Measurement (Three-Phase)/1 -> P/1
  Power Measurement (Three-Phase)/2 -> Q/1

== system ET3036TU_model_library_2021b/Bus Meassurement /Power Meassurement/phasor ==
  V : Inport
  I : Inport  Port=2
  "Power (3ph, Phasor)" : spsPower3phPhasorLib/Power (3ph, Phasor)
      settings: SourceProductBaseCode=PS
  P : Outport
  Q : Outport  Port=2
  wires:
  V/1 -> "Power (3ph, Phasor)"/1
  I/1 -> "Power (3ph, Phasor)"/2
  "Power (3ph, Phasor)"/1 -> P/1
  "Power (3ph, Phasor)"/2 -> Q/1

== system ET3036TU_model_library_2021b/Energy Storage/Battery over charging// discharging Protection/Over Charging Protection ==
  SOC (%) : Inport
  Pref : Inport  Port=2
  Constant1 : Constant  Value=ovrchargpro
  Constant2 : Constant  Value=UpChrgLim
  Display4 : Display
  GreaterThan : RelationalOperator  OutDataTypeStr=boolean  RndMeth=Simplest
  GreaterThan1 : RelationalOperator  Operator=<  OutDataTypeStr=boolean  RndMeth=Simplest
  Logical Operator : Logic  AllPortsSameDT=off  OutDataTypeStr=boolean
  MATLAB Function : MATLAB Function  TreatAsAtomicUnit=on
  Switch : Switch  Criteria=u2 ~= 0
  Zero : Constant  Value=0  OutDataTypeStr=Inherit: Inherit via back propagation
  Zero1 : Constant  Value=0  OutDataTypeStr=Inherit: Inherit via back propagation
  wires:
  Zero1/1 -> Switch/3
  Constant1/1 -> Switch/2
  Switch/1 -> MATLAB Function/1(u)
  Zero/1 -> GreaterThan1/2
  SOC (%)/1 -> GreaterThan/1
  GreaterThan1/1 -> Logical Operator/2
  Constant2/1 -> GreaterThan/2
  Logical Operator/1 -> Switch/1
  GreaterThan/1 -> Logical Operator/1, Display4/1
  Pref/1 -> GreaterThan1/1
